simulink model "RealModel"  (R2023b)
settings: Solver=VariableStepAuto  StartTime=0.0  StopTime=3600*50  RelTol=1e-3
undefined symbols (not defined in the file): magnitude
settings Model: Creator=ant  LastModifiedBy=ant

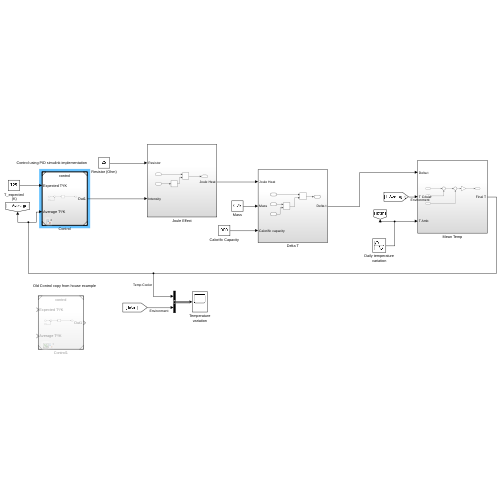
[thumbnail: Simulink's stored preview of the top-level diagram]
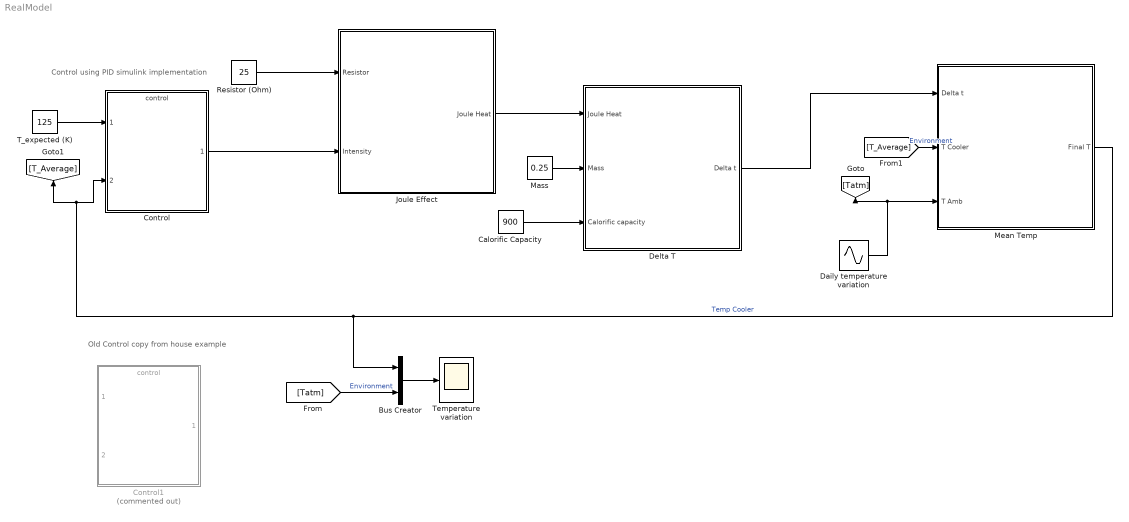
== system RealModel ==
  note: Control using PID simulink implementation
  note: Old Control copy from house example
  Bus Creator : BusCreator  Inputs=2
  Calorific Capacity : Constant  Value=900
  Control : ModelReference  ModelNameDialog=control.slx  SimulationMode=Normal  ModelReferenceVersion=1.5
  Control1 : ModelReference  Commented=on  ModelNameDialog=control.slx  SimulationMode=Normal  ModelReferenceVersion=1.4
  Daily temperature variation : Sin  Amplitude=0  Bias=120  Frequency=2*pi/(12*3600)  SampleTime=0
  Delta T : Subsystem
  Joule Effect : Subsystem
  Mass : Constant  Value=0.25
  Mean Temp : Subsystem
  Resistor (Ohm) : Constant  Value=25
  T_expected (K) : Constant  Value=125
  Temperature variation : Scope
  wires:
  T_expected (K)/1 -> Control/1
  Daily temperature variation/1 -> Mean Temp/3(T Amb), [Tatm]
  Joule Effect/1(Joule Heat) -> Delta T/1(Joule Heat)
  Delta T/1(Delta t) -> Mean Temp/1(Delta t)
  Resistor (Ohm)/1 -> Joule Effect/1(Resistor)
  Mass/1 -> Delta T/2(Mass)
  Calorific Capacity/1 -> Delta T/3(Calorific capacity)
  [Tatm] -> Bus Creator/2  "Environment"
  Mean Temp/1(Final T) -> Bus Creator/1, [T_Average], Control/2  "Temp Cooler"
  Bus Creator/1 -> Temperature variation/1
  [T_Average] -> Mean Temp/2(T Cooler)  "Environment"
  Control/1 -> Joule Effect/2(Intensity)

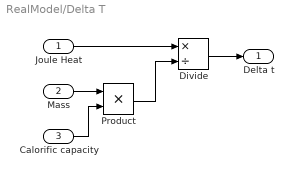
== system RealModel/Delta T ==
  Joule Heat : Inport
  Mass : Inport  Port=2
  Calorific capacity : Inport  Port=3
  Divide : Product  Inputs=*/
  Product : Product
  Delta t : Outport
  wires:
  Calorific capacity/1 -> Product/2
  Mass/1 -> Product/1
  Product/1 -> Divide/2
  Joule Heat/1 -> Divide/1
  Divide/1 -> Delta t/1

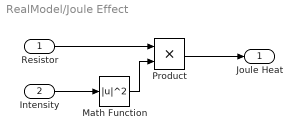
== system RealModel/Joule Effect ==
  Resistor : Inport
  Intensity : Inport  Port=2
  Math Function : Math  Operator=magnitude^2
  Product : Product
  Joule Heat : Outport
  wires:
  Math Function/1 -> Product/2
  Intensity/1 -> Math Function/1
  Resistor/1 -> Product/1
  Product/1 -> Joule Heat/1

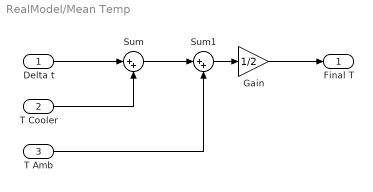
== system RealModel/Mean Temp ==
  Delta t : Inport
  T Cooler : Inport  Port=2
  T Amb : Inport  Port=3
  Gain : Gain  Gain=1/2
  Sum : Sum  Inputs=|++
  Sum1 : Sum  Inputs=|++
  Final T : Outport
  wires:
  Delta t/1 -> Sum/1
  T Cooler/1 -> Sum/2
  Sum/1 -> Sum1/1
  T Amb/1 -> Sum1/2
  Gain/1 -> Final T/1
  Sum1/1 -> Gain/1
